simulink model "parallel_modules_2_parasitic"  (R2023b)
settings: Solver=FixedStepDiscrete  StartTime=0.0  StopTime=Tfinal  FixedStep=SampleTime  RelTol=1e-3
InitFcn:
  | param
values from neighbouring files (symbols this model uses):
  ffund = 10    [param.m]
  Lload1 = 500e-6    (= 0.0005)    [param.m]
  ModulationIndex1 = 0.9    [param.m]
  Rload1 = 5    [param.m]
  SampleTime = 1e-6    (= 1e-06)    [param.m]
  Vdc = 50    [param.m]
libraries: simulink x7, spsGroundLib x6, spsMosfetLib x6, spsSeriesRLCBranchLib x4, spsVoltageMeasurementLib x4, spsCurrentMeasurementLib x4, spsDCVoltageSourceLib x1, spsTriangleGeneratorLib x1, BoomBox x1, sps_lib x1
settings Model: Creator=enes_  LastModifiedBy=enesa
settings SolverCC: AlgebraicLoopSolver=TrustRegion
settings DataIOCC: ReturnWorkspaceOutputs=off
settings DebuggingCC: UnconnectedInputMsg=warning  UnconnectedOutputMsg=warning  UnconnectedLineMsg=warning  ArithmeticOperatorsInVariantConditions=warning
settings ModelReferenceCC: EnableRefExpFcnMdlSchedulingChecks=on
settings SFSimCC: SimUseLocalCustomCode=off  CustomCodeUndefinedFunction=UseInterfaceOnly
settings RTWCC: RTWUseLocalCustomCode=off

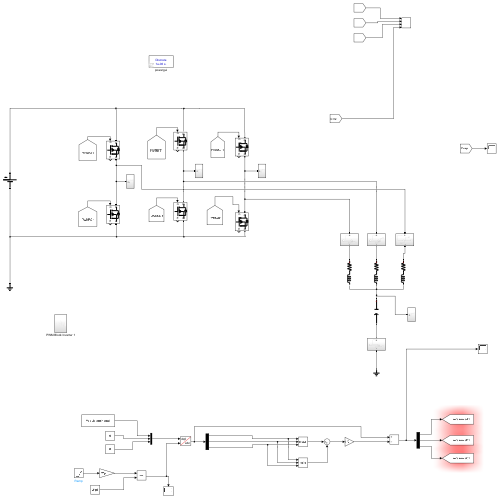
[thumbnail: Simulink's stored preview of the top-level diagram]
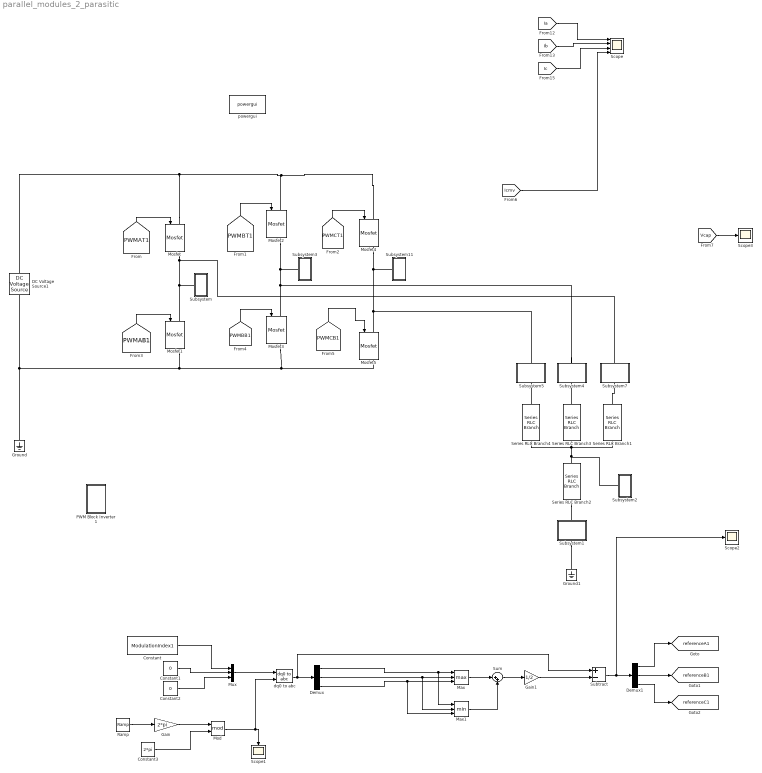
== system parallel_modules_2_parasitic ==
  Constant : Constant  Value=ModulationIndex1
  Constant1 : Constant  Value=0
  Constant2 : Constant  Value=0
  Constant3 : Constant  Value=2*pi
  DC Voltage Source1 : spsDCVoltageSourceLib/DC Voltage Source  Amplitude=Vdc  Measurements=None
  Demux : Demux  Outputs=3
  Demux1 : Demux  Outputs=3
  Gain : Gain  Gain=2*pi
  Gain1 : Gain  Gain=1/2
  Ground : spsGroundLib/Ground  LConnTagsString=a
  Ground1 : spsGroundLib/Ground  LConnTagsString=a
  Max : MinMax  Function=max  Inputs=3
  Max1 : MinMax  Inputs=3
  Mod : Math  Operator=mod
  Mosfet{,1..5} (6 alike) : spsMosfetLib/Mosfet  Ron=0.1  Lon=0  Rd=0.01  Vfd=0  IC=0  Rs=1e5  Cs=inf  Measurements=on
  Mux : Mux  Inputs=3
  PWM Block Inverter 1 : Subsystem
  Ramp : simulink/Sources/Ramp  slope=ffund  start=0  InitialOutput=0
  Scope : Scope  NumInputPorts=4
  Scope1 : Scope
  Scope2 : Scope
  Scope3 : Scope
  Series RLC Branch1 : spsSeriesRLCBranchLib/Series RLC Branch  LConnTagsString=__new0  RConnTagsString=__new0  BranchType=RL  Resistance=Rload1  Inductance=Lload1  SetiL0=off  InitialCurrent=0  Capacitance=1e-6  Setx0=off  InitialVoltage=0  Measurements=None
  Series RLC Branch2 : spsSeriesRLCBranchLib/Series RLC Branch  LConnTagsString=__new0  RConnTagsString=__new0  BranchType=C  Resistance=Rload1  Inductance=Lload1  SetiL0=off  InitialCurrent=0  Capacitance=10e-9  Setx0=off  InitialVoltage=0  Measurements=None
  Series RLC Branch3 : spsSeriesRLCBranchLib/Series RLC Branch  LConnTagsString=__new0  RConnTagsString=__new0  BranchType=RL  Resistance=Rload1  Inductance=Lload1  SetiL0=off  InitialCurrent=0  Capacitance=1e-6  Setx0=off  InitialVoltage=0  Measurements=None
  Series RLC Branch4 : spsSeriesRLCBranchLib/Series RLC Branch  LConnTagsString=__new0  RConnTagsString=__new0  BranchType=RL  Resistance=Rload1  Inductance=Lload1  SetiL0=off  InitialCurrent=0  Capacitance=1e-6  Setx0=off  InitialVoltage=0  Measurements=None
  Subsystem : Subsystem
  Subsystem1 : Subsystem
  Subsystem11 : Subsystem
  Subsystem2 : Subsystem
  Subsystem3 : Subsystem
  Subsystem4 : Subsystem
  Subsystem5 : Subsystem
  Subsystem7 : Subsystem
  Subtract : Sum  Inputs=+-
  Sum : Sum  Inputs=|++
  dq0 to abc : BoomBox/Transformations/dq0 to abc  KBID=kb0602
      settings: SourceProductName=imperix blockset
  powergui : sps_lib/powergui  Priority=1  SimulationMode=Discrete  SampleTime=SampleTime  frequency=60  Iterations=50  frequencyindice=0  Pbase=100e6  ErrMax=1e-4  UnitsV=kV  UnitsW=MW  buscounter=0  FunctionMessages=off  echomessages=off  EnableUseOfTLC=off  CurrentSourceSwitches=off  DisableSnubberDevices=off  DisableRonSwitches=off  DisableVfSwitches=off  DisplayEquations=off  AutomaticDiscreteSolvers=off  SolverType=Tustin/Backward Euler (TBE)  Interpol=off  ExternalGateDelay=off  methode=off  Ts=100  x0status=blocks  SPID=off  SwTol=0  HookPort=off  NonlinearTolerance=1e-4  nMaxIteration=100  ContinueOnMaxIteration=off  RestoreLinks=warning  ResistiveCurrentMeasurement=off  Frange=[0:2:500]  Ylog=off  Xlog=on  ShowGrid=off  save=off  variable=ZData  structure=0  ZoomFFT=off  StartTime=0.0  cycles=1  DisplayStyle=1  fundamental=60  FreqAxis=off  MaxFrequency=1000  frequencyindicesteady=1  RmsSteady=1  display=off
  tag scope: referenceA1=global, referenceB1=global, referenceC1=global
  wires:
  [PWMBB1] -> Mosfet3/1
  [PWMCB1] -> Mosfet5/1
  [PWMAB1] -> Mosfet1/1
  [PWMBT1] -> Mosfet2/1
  [PWMCT1] -> Mosfet4/1
  [PWMAT1] -> Mosfet/1
  Constant/1 -> Mux/1
  Constant1/1 -> Mux/2
  Constant2/1 -> Mux/3
  Mux/1 -> dq0 to abc/1
  Constant3/1 -> Mod/2
  Mod/1 -> Scope1/1, dq0 to abc/2
  dq0 to abc/1 -> Subtract/1, Demux/1
  Gain/1 -> Mod/1
  Ramp/1 -> Gain/1
  Demux/1 -> Max1/1, Max/1
  Demux/2 -> Max1/2, Max/2
  Demux/3 -> Max1/3, Max/3
  [Ia] -> Scope/1
  [Ib] -> Scope/2
  [Ic] -> Scope/3
  [Icmv] -> Scope/4
  Max/1 -> Sum/1
  Max1/1 -> Sum/2
  Sum/1 -> Gain1/1
  Gain1/1 -> Subtract/2
  Subtract/1 -> Scope2/1, Demux1/1
  Demux1/1 -> [referenceA1]
  Demux1/2 -> [referenceB1]
  Demux1/3 -> [referenceC1]
  [Vcap] -> Scope3/1
  connections:
  Series RLC Branch3/LConn1 -- Subsystem4/LConn1
  Series RLC Branch4/LConn1 -- Subsystem5/LConn1
  Mosfet2/RConn1 -- Subsystem3/LConn1 -- Subsystem4/RConn1 -- Mosfet3/LConn1
  Mosfet4/RConn1 -- Subsystem11/LConn1 -- Subsystem5/RConn1 -- Mosfet5/LConn1
  Mosfet/RConn1 -- Subsystem7/RConn1 -- Subsystem/LConn1 -- Mosfet1/LConn1
  Mosfet/LConn1 -- DC Voltage Source1/RConn1 -- Mosfet2/LConn1 -- Mosfet4/LConn1
  Series RLC Branch1/LConn1 -- Subsystem7/LConn1
  Mosfet1/RConn1 -- Mosfet3/RConn1 -- Mosfet5/RConn1 -- DC Voltage Source1/LConn1 -- Ground/LConn1
  Series RLC Branch4/RConn1 -- Subsystem2/LConn1 -- Series RLC Branch2/LConn1 -- Series RLC Branch1/RConn1 -- Series RLC Branch3/RConn1
  Subsystem1/LConn1 -- Ground1/LConn1
  Series RLC Branch2/RConn1 -- Subsystem1/RConn1

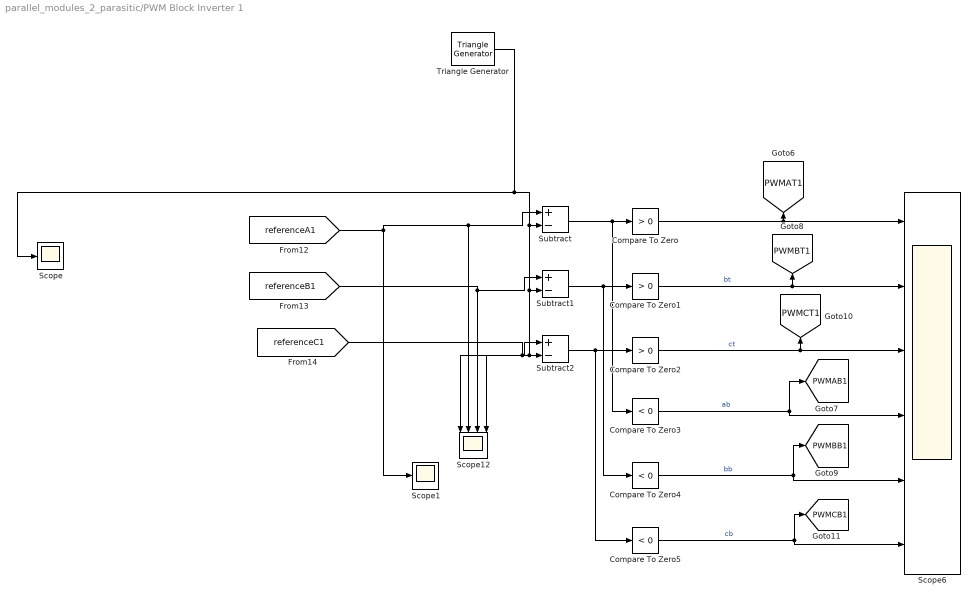
== system parallel_modules_2_parasitic/PWM Block Inverter 1 ==
  Compare To Zero : simulink/Logic and Bit Operations/Compare To Zero  relop=>  OutDataTypeStr=boolean
  Compare To Zero1 : simulink/Logic and Bit Operations/Compare To Zero  relop=>  OutDataTypeStr=boolean
  Compare To Zero2 : simulink/Logic and Bit Operations/Compare To Zero  relop=>  OutDataTypeStr=boolean
  Compare To Zero3 : simulink/Logic and Bit Operations/Compare To Zero  relop=<  OutDataTypeStr=boolean
  Compare To Zero4 : simulink/Logic and Bit Operations/Compare To Zero  relop=<  OutDataTypeStr=boolean
  Compare To Zero5 : simulink/Logic and Bit Operations/Compare To Zero  relop=<  OutDataTypeStr=boolean
  Scope : Scope
  Scope1 : Scope
  Scope12 : Scope  NumInputPorts=4
  Scope6 : Scope  NumInputPorts=6
  Subtract : Sum  Inputs=+-
  Subtract1 : Sum  Inputs=+-
  Subtract2 : Sum  Inputs=+-
  Triangle Generator : spsTriangleGeneratorLib/Triangle Generator  Freq=fsw  Phase=0  Ts=SampleTime
  tag scope: PWMAB1=global, PWMAT1=global, PWMBB1=global, PWMBT1=global, PWMCB1=global, PWMCT1=global
  wires:
  Compare To Zero2/1 -> [PWMCT1], Scope6/3  "ct"
  [referenceB1] -> Subtract1/1, Scope12/3
  Subtract2/1 -> Compare To Zero5/1, Compare To Zero2/1
  [referenceA1] -> Subtract/1, Scope12/2, Scope1/1
  Subtract1/1 -> Compare To Zero4/1, Compare To Zero1/1
  Triangle Generator/1 -> Scope12/1, Subtract2/2, Subtract1/2, Subtract/2, Scope/1
  Compare To Zero/1 -> Scope6/1, [PWMAT1]
  Subtract/1 -> Compare To Zero3/1, Compare To Zero/1
  Compare To Zero1/1 -> [PWMBT1], Scope6/2  "bt"
  Compare To Zero5/1 -> [PWMCB1], Scope6/6  "cb"
  Compare To Zero4/1 -> [PWMBB1], Scope6/5  "bb"
  [referenceC1] -> Scope12/4, Subtract2/1
  Compare To Zero3/1 -> [PWMAB1], Scope6/4  "ab"

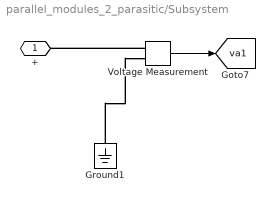
== system parallel_modules_2_parasitic/Subsystem ==
  Ground1 : spsGroundLib/Ground  LConnTagsString=a
  Voltage Measurement : spsVoltageMeasurementLib/Voltage Measurement  PhasorSimulation=off  OutputType=Complex  PSBequivalent=0
  + : PMIOPort  Side=Left
  tag scope: va1=global
  wires:
  Voltage Measurement/1 -> [va1]
  connections:
  Voltage Measurement/LConn1 -- +/RConn1
  Ground1/LConn1 -- Voltage Measurement/LConn2

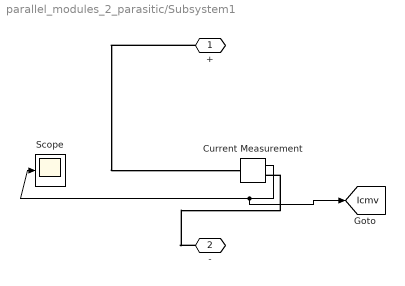
== system parallel_modules_2_parasitic/Subsystem1 ==
  Current Measurement : spsCurrentMeasurementLib/Current Measurement  PhasorSimulation=off  OutputType=Complex  PSBequivalent=0
  Scope : Scope
  + : PMIOPort  Side=Right
  - : PMIOPort  Port=2  Side=Left
  tag scope: Icmv=global
  wires:
  Current Measurement/1 -> Scope/1, [Icmv]
  connections:
  +/RConn1 -- Current Measurement/LConn1
  -/RConn1 -- Current Measurement/RConn1

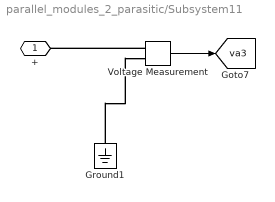
== system parallel_modules_2_parasitic/Subsystem11 ==
  Ground1 : spsGroundLib/Ground  LConnTagsString=a
  Voltage Measurement : spsVoltageMeasurementLib/Voltage Measurement  PhasorSimulation=off  OutputType=Complex  PSBequivalent=0
  + : PMIOPort  Side=Left
  tag scope: va3=global
  wires:
  Voltage Measurement/1 -> [va3]
  connections:
  Voltage Measurement/LConn1 -- +/RConn1
  Ground1/LConn1 -- Voltage Measurement/LConn2

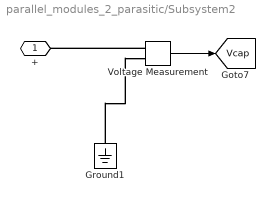
== system parallel_modules_2_parasitic/Subsystem2 ==
  Ground1 : spsGroundLib/Ground  LConnTagsString=a
  Voltage Measurement : spsVoltageMeasurementLib/Voltage Measurement  PhasorSimulation=off  OutputType=Complex  PSBequivalent=0
  + : PMIOPort  Side=Left
  tag scope: Vcap=global
  wires:
  Voltage Measurement/1 -> [Vcap]
  connections:
  Voltage Measurement/LConn1 -- +/RConn1
  Ground1/LConn1 -- Voltage Measurement/LConn2

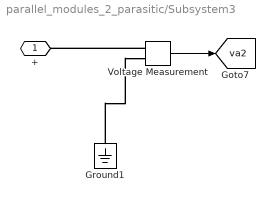
== system parallel_modules_2_parasitic/Subsystem3 ==
  Ground1 : spsGroundLib/Ground  LConnTagsString=a
  Voltage Measurement : spsVoltageMeasurementLib/Voltage Measurement  PhasorSimulation=off  OutputType=Complex  PSBequivalent=0
  + : PMIOPort  Side=Left
  tag scope: va2=global
  wires:
  Voltage Measurement/1 -> [va2]
  connections:
  Voltage Measurement/LConn1 -- +/RConn1
  Ground1/LConn1 -- Voltage Measurement/LConn2

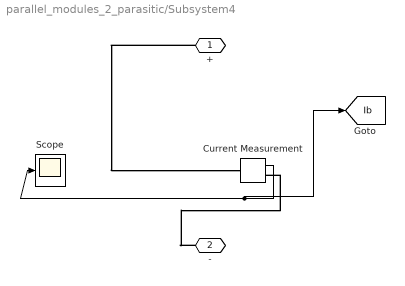
== system parallel_modules_2_parasitic/Subsystem4 ==
  Current Measurement : spsCurrentMeasurementLib/Current Measurement  PhasorSimulation=off  OutputType=Complex  PSBequivalent=0
  Scope : Scope
  + : PMIOPort  Side=Right
  - : PMIOPort  Port=2  Side=Left
  tag scope: Ib=global
  wires:
  Current Measurement/1 -> [Ib], Scope/1
  connections:
  +/RConn1 -- Current Measurement/LConn1
  -/RConn1 -- Current Measurement/RConn1

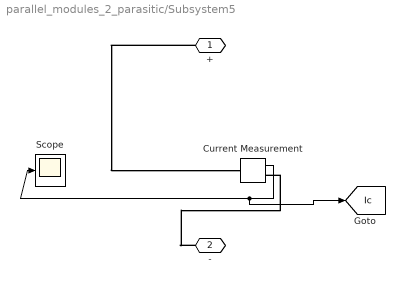
== system parallel_modules_2_parasitic/Subsystem5 ==
  Current Measurement : spsCurrentMeasurementLib/Current Measurement  PhasorSimulation=off  OutputType=Complex  PSBequivalent=0
  Scope : Scope
  + : PMIOPort  Side=Right
  - : PMIOPort  Port=2  Side=Left
  tag scope: Ic=global
  wires:
  Current Measurement/1 -> Scope/1, [Ic]
  connections:
  +/RConn1 -- Current Measurement/LConn1
  -/RConn1 -- Current Measurement/RConn1

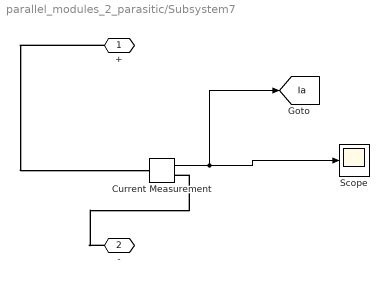
== system parallel_modules_2_parasitic/Subsystem7 ==
  Current Measurement : spsCurrentMeasurementLib/Current Measurement  PhasorSimulation=off  OutputType=Complex  PSBequivalent=0
  Scope : Scope
  + : PMIOPort  Side=Right
  - : PMIOPort  Port=2  Side=Left
  tag scope: Ia=global
  wires:
  Current Measurement/1 -> [Ia], Scope/1
  connections:
  +/RConn1 -- Current Measurement/LConn1
  -/RConn1 -- Current Measurement/RConn1
